simulink model "SSW345MidtermTwo"  (R2024b)
settings: Solver=VariableStepAuto  StartTime=0.0  StopTime=10.0  RelTol=1e-3
libraries: simulink x10
settings Model: Creator=ferbe  LastModifiedBy=ferbe

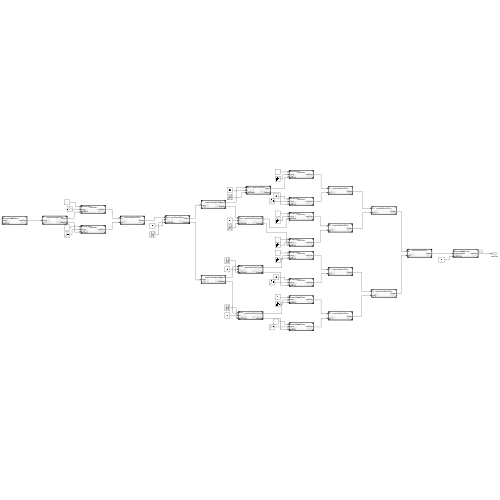
[thumbnail: Simulink's stored preview of the top-level diagram]
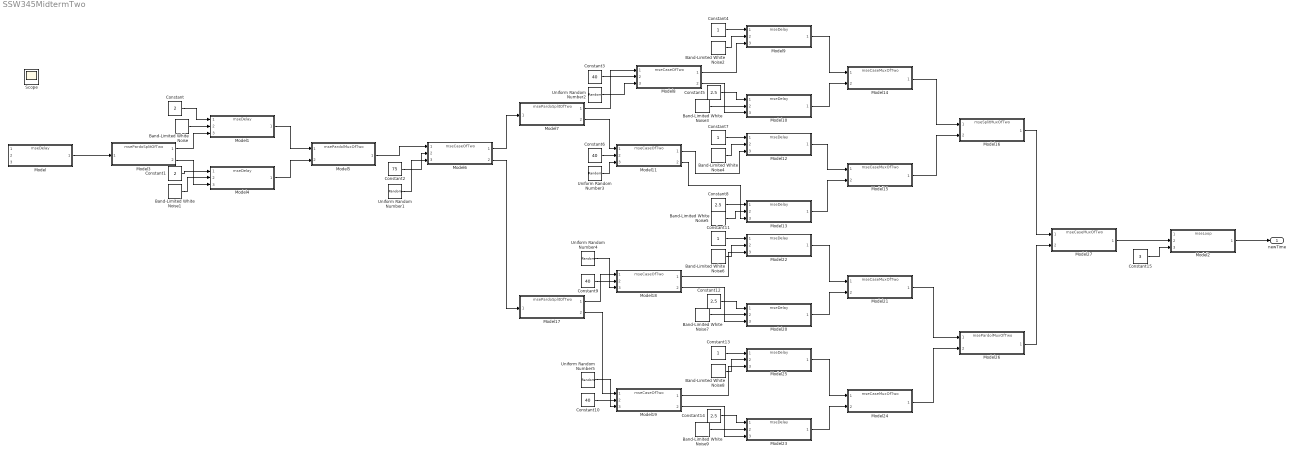
== system SSW345MidtermTwo ==
  Band-Limited White Noise{,1..9} (10 alike) : simulink/Sources/Band-Limited White Noise  Cov=[0.1]  Ts=0.1  seed=[23341]
  Constant : Constant  Value=2
  Constant1 : Constant  Value=2
  Constant{3,6,9..10} (4 alike) : Constant  Value=40
  Constant{4,7,11,13} (4 alike) : Constant
  Constant{5,8,12,14} (4 alike) : Constant  Value=2.5
  Constant15 : Constant  Value=3
  Constant2 : Constant  Value=75
  Model{,1,4,9..10,12..13,20,22..23,25} (11 alike) : ModelReference  ModelNameDialog=mseDelay.slx  SimulationMode=Normal  ModelReferenceVersion=3.7
  Model{6,8,11,18..19} (5 alike) : ModelReference  ModelNameDialog=mseCaseOfTwo.slx  SimulationMode=Normal  ModelReferenceVersion=3.9
  Model{14..15,21,24,27} (5 alike) : ModelReference  ModelNameDialog=mseCaseMuxOfTwo.slx  SimulationMode=Normal  ModelReferenceVersion=3.0
  Model16 : ModelReference  ModelNameDialog=mseSplitMuxOfTwo.slx  SimulationMode=Normal  ModelReferenceVersion=3.2
  Model17 : ModelReference  ModelNameDialog=msePardoSplitOfTwo.slx  SimulationMode=Normal  ModelReferenceVersion=3.2
  Model2 : ModelReference  ModelNameDialog=mseLoop.slx  SimulationMode=Normal  ModelReferenceVersion=3.1
  Model26 : ModelReference  ModelNameDialog=msePardolMuxOfTwo.slx  SimulationMode=Normal  ModelReferenceVersion=3.3
  Model3 : ModelReference  ModelNameDialog=msePardoSplitOfTwo.slx  SimulationMode=Normal  ModelReferenceVersion=3.2
  Model5 : ModelReference  ModelNameDialog=msePardolMuxOfTwo.slx  SimulationMode=Normal  ModelReferenceVersion=3.3
  Model7 : ModelReference  ModelNameDialog=msePardoSplitOfTwo.slx  SimulationMode=Normal  ModelReferenceVersion=3.2
  Uniform Random Number{1..5} (5 alike) : UniformRandomNumber  Minimum=0  Maximum=100  SampleTime=0.1
  newTime : Outport
  Scope : Scope
  wires:
  Model/1 -> Model3/1
  Model3/1 -> Model1/3
  Model3/2 -> Model4/3
  Constant/1 -> Model1/1
  Band-Limited White Noise/1 -> Model1/2
  Constant1/1 -> Model4/1
  Band-Limited White Noise1/1 -> Model4/2
  Model4/1 -> Model5/2
  Model1/1 -> Model5/1
  Model5/1 -> Model6/1
  Constant2/1 -> Model6/2
  Uniform Random Number1/1 -> Model6/3
  Model6/1 -> Model7/1
  Model7/1 -> Model8/1
  Constant3/1 -> Model8/2
  Uniform Random Number2/1 -> Model8/3
  Model8/1 -> Model9/3
  Band-Limited White Noise2/1 -> Model9/2
  Constant4/1 -> Model9/1
  Model8/2 -> Model10/3
  Band-Limited White Noise3/1 -> Model10/2
  Constant5/1 -> Model10/1
  Model11/2 -> Model13/3
  Constant8/1 -> Model13/1
  Band-Limited White Noise4/1 -> Model12/2
  Constant6/1 -> Model11/2
  Model11/1 -> Model12/3
  Constant7/1 -> Model12/1
  Uniform Random Number3/1 -> Model11/3
  Band-Limited White Noise5/1 -> Model13/2
  Model7/2 -> Model11/1
  Model9/1 -> Model14/1
  Model10/1 -> Model14/2
  Model12/1 -> Model15/1
  Model13/1 -> Model15/2
  Model14/1 -> Model16/1
  Model15/1 -> Model16/2
  Model6/2 -> Model17/1
  Model17/1 -> Model18/1
  Constant9/1 -> Model18/2
  Uniform Random Number4/1 -> Model18/3
  Uniform Random Number5/1 -> Model19/3
  Constant10/1 -> Model19/2
  Model17/2 -> Model19/1
  Model18/1 -> Model22/3
  Model18/2 -> Model20/3
  Constant12/1 -> Model20/1
  Band-Limited White Noise7/1 -> Model20/2
  Band-Limited White Noise6/1 -> Model22/2
  Constant11/1 -> Model22/1
  Model22/1 -> Model21/1
  Model20/1 -> Model21/2
  Model19/1 -> Model25/3
  Model19/2 -> Model23/3
  Constant14/1 -> Model23/1
  Band-Limited White Noise9/1 -> Model23/2
  Band-Limited White Noise8/1 -> Model25/2
  Constant13/1 -> Model25/1
  Model25/1 -> Model24/1
  Model23/1 -> Model24/2
  Model21/1 -> Model26/1
  Model24/1 -> Model26/2
  Model16/1 -> Model27/1
  Model26/1 -> Model27/2
  Model27/1 -> Model2/2
  Constant15/1 -> Model2/3
  Model2/1 -> newTime/1
